simulink model "VCU_SW_2020"  (R2020b)
settings: Solver=FixedStepDiscrete  StartTime=0.0  StopTime=inf  FixedStep=1e-2  RelTol=1e-3
PreLoadFcn:
  | RTWConfigurationCB('preloadfcn', bdroot);
InitFcn:
  | loadvar_ttc500
undefined symbols (not defined in the file): BrkPedalTypes, CabMovModeTypes, cFuseTempSensAcc_X, cFuseTempSensAcc_Y, cFuseTempSensVal_X, cFuseTempSensVal_Y, cTMSTempSensVal_X, cTMSTempSensVal_Y, cTransferCaseSpeedRatio, diag_state, DoorsPositionTypes, dP_filter_Y, DriverOccClassSystemTypes, ErrorValueTypes, fatal_error_callback, IO_ADC_NO_RANGE, LadderStatusTypes, pAnalogCabRotSensAcc, pAnalogCabRotSensMaxVolt, pAnalogCabRotSensMinVolt, pAnalogCabRotSensRange, pAnalogCabRotSensZeroVolt, pBrkActivePress, pCabTiltSensAcc, pCabTiltSensMaxCur, pCabTiltSensMinCur, pDistanceCorrection, pECANManual_BPNEnable, pECANManual_BPNEnabler_Flag, pFilterSensAccRes, pHDirMaxDiffFrq, pHDirSensHighLvl, pHDirSensLowLvl, pMainGearRatio, pMaxFilterSensRes, pMaxFirstPedalSensValue, pMaxFuseTempSensRes, pMaxPressLoss, pMaxPressSensCurrent, pMaxPressValue, pMaxPressValueHydMotAndPump, pMaxPressValueParkDrain, pMaxSecondPedalSensValue, pMaxTempSensVoltage, pMaxTempValue, pMaxTMSTempSensRes, pMinFilterSensRes, pMinFirstPedalSensValue, pMinFuseTempSensRes, pMinPressLoss, pMinPressSensCurrent, pMinPressValue, pMinSecondPedalSensValue, pMinTempSensVoltage, pMinTempValue, pMinTMSTempSensRes, pMotorRingTeethNum, pPedalSensAccuracyPct, pPedalSensAccuracyVolt, pPressLossTreshhold ... (+20)
libraries: TTlibrary x270, canmsglib x127, simulink x88
(part 3 of 17)

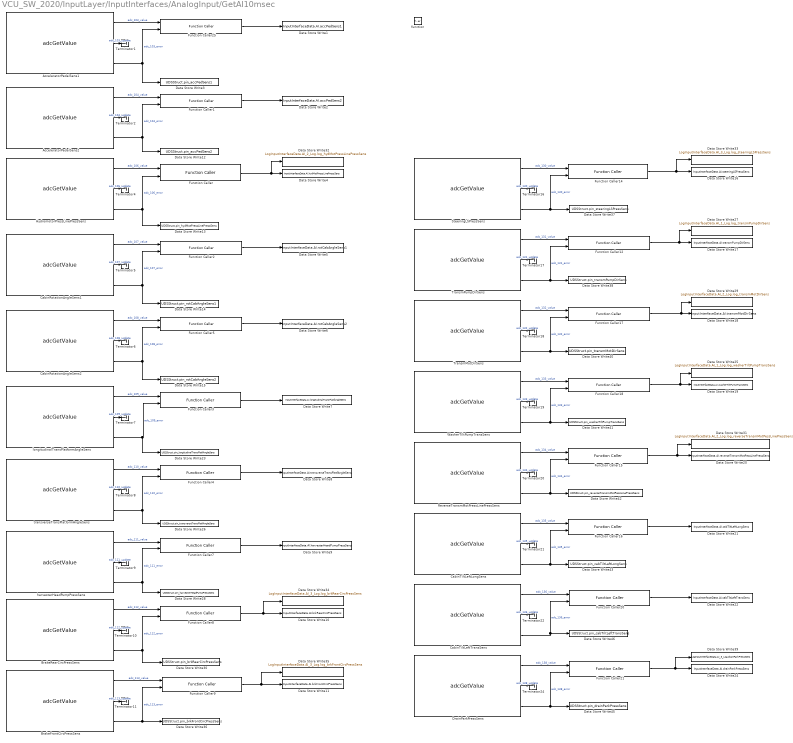
== system VCU_SW_2020/InputLayer/InputInterfaces/AnalogInput/GetAI10msec ==
  function : TriggerPort  TriggerType=function-call  VariantControl=Variant
  AcceleratorPedalSens1 : TTlibrary/ADC/adcGetValue  adc_channel=IO_ADC_00  types=IO_ADC_RATIOMETRIC  range=IO_ADC_NO_RANGE  pupd=IO_ADC_NO_PULL  sensor_supply=IO_SENSOR_SUPPLY_1  safety_conf=off  adc_val_lower=4  adc_val_upper=4  redundant_channel=IO_ADC_08  io_error=on  sample_time=-1
      settings: SourceProductName=TT control 500 series
  AcceleratorPedalSens2 : TTlibrary/ADC/adcGetValue  adc_channel=IO_ADC_02  types=IO_ADC_RATIOMETRIC  range=IO_ADC_NO_RANGE  pupd=IO_ADC_NO_PULL  sensor_supply=IO_SENSOR_SUPPLY_1  safety_conf=off  adc_val_lower=4  adc_val_upper=4  redundant_channel=IO_ADC_08  io_error=on  sample_time=-1
      settings: SourceProductName=TT control 500 series
  BrakeFrontCircPressSens : TTlibrary/ADC/adcGetValue  adc_channel=IO_ADC_20  types=IO_ADC_CURRENT  range=IO_ADC_NO_RANGE  pupd=IO_ADC_NO_PULL  sensor_supply=IO_PIN_NONE  safety_conf=off  adc_val_lower=4  adc_val_upper=4  redundant_channel=IO_ADC_08  io_error=on  sample_time=-1
      settings: SourceProductName=TT control 500 series
  BrakeRearCircPressSens : TTlibrary/ADC/adcGetValue  adc_channel=IO_ADC_18  types=IO_ADC_CURRENT  range=IO_ADC_NO_RANGE  pupd=IO_ADC_NO_PULL  sensor_supply=IO_PIN_NONE  safety_conf=off  adc_val_lower=4  adc_val_upper=4  redundant_channel=IO_ADC_08  io_error=on  sample_time=-1
      settings: SourceProductName=TT control 500 series
  CabinRotationAngleSens1 : TTlibrary/ADC/adcGetValue  adc_channel=IO_ADC_08  types=IO_ADC_RATIOMETRIC  range=IO_ADC_RANGE_5V  pupd=IO_ADC_NO_PULL  sensor_supply=IO_SENSOR_SUPPLY_2  safety_conf=off  adc_val_lower=4  adc_val_upper=4  redundant_channel=IO_ADC_08  io_error=on  sample_time=-1
      settings: SourceProductName=TT control 500 series
  CabinRotationAngleSens2 : TTlibrary/ADC/adcGetValue  adc_channel=IO_ADC_10  types=IO_ADC_RATIOMETRIC  range=IO_ADC_RANGE_5V  pupd=IO_ADC_NO_PULL  sensor_supply=IO_SENSOR_SUPPLY_2  safety_conf=off  adc_val_lower=4  adc_val_upper=4  redundant_channel=IO_ADC_08  io_error=on  sample_time=-1
      settings: SourceProductName=TT control 500 series
  CabinTiltLeftLongSens : TTlibrary/ADC/adcGetValue  adc_channel=IO_ADC_17  types=IO_ADC_CURRENT  range=IO_ADC_NO_RANGE  pupd=IO_ADC_NO_PULL  sensor_supply=IO_PIN_NONE  safety_conf=off  adc_val_lower=4  adc_val_upper=4  redundant_channel=IO_ADC_08  io_error=on  sample_time=-1
      settings: SourceProductName=TT control 500 series
  CabinTiltLeftTransSens : TTlibrary/ADC/adcGetValue  adc_channel=IO_ADC_19  types=IO_ADC_CURRENT  range=IO_ADC_NO_RANGE  pupd=IO_ADC_NO_PULL  sensor_supply=IO_PIN_NONE  safety_conf=off  adc_val_lower=4  adc_val_upper=4  redundant_channel=IO_ADC_08  io_error=on  sample_time=-1
      settings: SourceProductName=TT control 500 series
  Data Store Write1 : DataStoreWrite  DataStoreName=InputInterfaceData  DataStoreElements=InputInterfaceData.AI.accPedSens1
  Data Store Write10 : DataStoreWrite  DataStoreName=InputInterfaceData  DataStoreElements=InputInterfaceData.AI.brkRearCircPressSens
  Data Store Write11 : DataStoreWrite  DataStoreName=InputInterfaceData  DataStoreElements=InputInterfaceData.AI.brkFrontCircPressSens
  Data Store Write12 : DataStoreWrite  DataStoreName=UDSStruct  DataStoreElements=UDSStruct.pin_accPedSens2
  Data Store Write13 : DataStoreWrite  DataStoreName=UDSStruct  DataStoreElements=UDSStruct.pin_hydMotPressLinePressSens
  Data Store Write14 : DataStoreWrite  DataStoreName=UDSStruct  DataStoreElements=UDSStruct.pin_rotCabAngleSens1
  Data Store Write15 : DataStoreWrite  DataStoreName=UDSStruct  DataStoreElements=UDSStruct.pin_rotCabAngleSens2
  Data Store Write16 : DataStoreWrite  DataStoreName=InputInterfaceData  DataStoreElements=InputInterfaceData.AI.steeringLSPressSens
  Data Store Write17 : DataStoreWrite  DataStoreName=InputInterfaceData  DataStoreElements=InputInterfaceData.AI.transmPumpDirSens
  Data Store Write18 : DataStoreWrite  DataStoreName=InputInterfaceData  DataStoreElements=InputInterfaceData.AI.transmMotDirSens
  Data Store Write19 : DataStoreWrite  DataStoreName=InputInterfaceData  DataStoreElements=InputInterfaceData.AI.washerTiltPumpTransSens
  Data Store Write2 : DataStoreWrite  DataStoreName=InputInterfaceData  DataStoreElements=InputInterfaceData.AI.accPedSens2
  Data Store Write20 : DataStoreWrite  DataStoreName=InputInterfaceData  DataStoreElements=InputInterfaceData.AI.reverseTransmMotPessLinePressSens
  Data Store Write21 : DataStoreWrite  DataStoreName=InputInterfaceData  DataStoreElements=InputInterfaceData.AI.cabTiltLeftLongSens
  Data Store Write22 : DataStoreWrite  DataStoreName=InputInterfaceData  DataStoreElements=InputInterfaceData.AI.cabTiltLeftTransSens
  Data Store Write23 : DataStoreWrite  DataStoreName=UDSStruct  DataStoreElements=UDSStruct.pin_longitudinalTransPlatfAngleSens
  Data Store Write24 : DataStoreWrite  DataStoreName=InputInterfaceData  DataStoreElements=InputInterfaceData.AI.drainParkPressSens
  Data Store Write25 : DataStoreWrite  DataStoreName=LogInputInterfaceData  DataStoreElements=LogInputInterfaceData.AI_1_Log.log_washerTiltPumpTransSens
  Data Store Write26 : DataStoreWrite  DataStoreName=UDSStruct  DataStoreElements=UDSStruct.pin_transverseTransPlatfAngleSens
  Data Store Write27 : DataStoreWrite  DataStoreName=LogInputInterfaceData  DataStoreElements=LogInputInterfaceData.AI_1_Log.log_transmPumpDirSens
  Data Store Write28 : DataStoreWrite  DataStoreName=UDSStruct  DataStoreElements=UDSStruct.pin_harvesterHeadPumpPressSens
  Data Store Write29 : DataStoreWrite  DataStoreName=LogInputInterfaceData  DataStoreElements=LogInputInterfaceData.AI_2_Log.log_transmMotDirSens
  Data Store Write3 : DataStoreWrite  DataStoreName=UDSStruct  DataStoreElements=UDSStruct.pin_accPedSens1
  Data Store Write30 : DataStoreWrite  DataStoreName=UDSStruct  DataStoreElements=UDSStruct.pin_brkRearCircPressSens
  Data Store Write31 : DataStoreWrite  DataStoreName=LogInputInterfaceData  DataStoreElements=LogInputInterfaceData.AI_2_Log.log_reverseTransmMotPessLinePressSens
  Data Store Write32 : DataStoreWrite  DataStoreName=LogInputInterfaceData  DataStoreElements=LogInputInterfaceData.AI_2_Log.log_hydMotPressLinePressSens
  Data Store Write33 : DataStoreWrite  DataStoreName=LogInputInterfaceData  DataStoreElements=LogInputInterfaceData.AI_3_Log.log_steeringLSPressSens
  Data Store Write34 : DataStoreWrite  DataStoreName=LogInputInterfaceData  DataStoreElements=LogInputInterfaceData.AI_3_Log.log_brkRearCircPressSens
  Data Store Write35 : DataStoreWrite  DataStoreName=LogInputInterfaceData  DataStoreElements=LogInputInterfaceData.AI_3_Log.log_brkFrontCircPressSens
  Data Store Write36 : DataStoreWrite  DataStoreName=UDSStruct  DataStoreElements=UDSStruct.pin_brkFrontCircPressSens
  Data Store Write37 : DataStoreWrite  DataStoreName=UDSStruct  DataStoreElements=UDSStruct.pin_steeringLSPressSens
  Data Store Write38 : DataStoreWrite  DataStoreName=UDSStruct  DataStoreElements=UDSStruct.pin_transmPumpDirSens
  Data Store Write39 : DataStoreWrite  DataStoreName=LogInputInterfaceData  DataStoreElements=LogInputInterfaceData.AI_3_Log.drainParkPressSens
  Data Store Write4 : DataStoreWrite  DataStoreName=InputInterfaceData  DataStoreElements=InputInterfaceData.AI.hydMotPressLinePressSens
  Data Store Write40 : DataStoreWrite  DataStoreName=UDSStruct  DataStoreElements=UDSStruct.pin_transmMotDirSens
  Data Store Write41 : DataStoreWrite  DataStoreName=UDSStruct  DataStoreElements=UDSStruct.pin_washerTiltPumpTransSens
  Data Store Write42 : DataStoreWrite  DataStoreName=UDSStruct  DataStoreElements=UDSStruct.pin_reverseTransmMotPessLinePressSens
  Data Store Write43 : DataStoreWrite  DataStoreName=UDSStruct  DataStoreElements=UDSStruct.pin_cabTiltLeftLongSens
  Data Store Write45 : DataStoreWrite  DataStoreName=UDSStruct  DataStoreElements=UDSStruct.pin_drainParkPressSens
  Data Store Write46 : DataStoreWrite  DataStoreName=UDSStruct  DataStoreElements=UDSStruct.pin_cabTiltLeftTransSens
  Data Store Write5 : DataStoreWrite  DataStoreName=InputInterfaceData  DataStoreElements=InputInterfaceData.AI.rotCabAngleSens1
  Data Store Write6 : DataStoreWrite  DataStoreName=InputInterfaceData  DataStoreElements=InputInterfaceData.AI.rotCabAngleSens2
  Data Store Write7 : DataStoreWrite  DataStoreName=InputInterfaceData  DataStoreElements=InputInterfaceData.AI.longitudinalTransPlatfAngleSens
  Data Store Write8 : DataStoreWrite  DataStoreName=InputInterfaceData  DataStoreElements=InputInterfaceData.AI.transverseTransPlatfAngleSens
  Data Store Write9 : DataStoreWrite  DataStoreName=InputInterfaceData  DataStoreElements=InputInterfaceData.AI.harvesterHeadPumpPressSens
  DrainParkPressSens : TTlibrary/ADC/adcGetValue  adc_channel=IO_ADC_23  types=IO_ADC_CURRENT  range=IO_ADC_NO_RANGE  pupd=IO_ADC_NO_PULL  sensor_supply=IO_PIN_NONE  safety_conf=off  adc_val_lower=4  adc_val_upper=4  redundant_channel=IO_ADC_08  io_error=on  sample_time=-1
      settings: SourceProductName=TT control 500 series
  Function Caller{,3..4,7..9,14..16,20..21} (11 alike) : FunctionCaller  FunctionPrototype=finalValue = convAICurrentData(rawValue,errorSts)  InputArgumentSpecifications=<Enter example>  OutputArgumentSpecifications=<Enter example>
  Function Caller{1..2,5,12,17..18,25} (7 alike) : FunctionCaller  FunctionPrototype=finalValue = convAIVoltageData(rawValue,errorSts)  InputArgumentSpecifications=<Enter example>  OutputArgumentSpecifications=<Enter example>
  HydromotorPressLinePressSens : TTlibrary/ADC/adcGetValue  adc_channel=IO_ADC_06  types=IO_ADC_CURRENT  range=IO_ADC_NO_RANGE  pupd=IO_ADC_NO_PULL  sensor_supply=IO_PIN_NONE  safety_conf=off  adc_val_lower=4  adc_val_upper=4  redundant_channel=IO_ADC_08  io_error=on  sample_time=-1
      settings: SourceProductName=TT control 500 series
  ReverseTransmMotPressLinePressSens : TTlibrary/ADC/adcGetValue  adc_channel=IO_ADC_15  types=IO_ADC_CURRENT  range=IO_ADC_NO_RANGE  pupd=IO_ADC_NO_PULL  sensor_supply=IO_PIN_NONE  safety_conf=off  adc_val_lower=4  adc_val_upper=4  redundant_channel=IO_ADC_08  io_error=on  sample_time=-1
      settings: SourceProductName=TT control 500 series
  SteeringLSPressSens : TTlibrary/ADC/adcGetValue  adc_channel=IO_ADC_07  types=IO_ADC_CURRENT  range=IO_ADC_NO_RANGE  pupd=IO_ADC_NO_PULL  sensor_supply=IO_PIN_NONE  safety_conf=off  adc_val_lower=4  adc_val_upper=4  redundant_channel=IO_ADC_08  io_error=on  sample_time=-1
      settings: SourceProductName=TT control 500 series
  Terminator{1..2,4..11,16..22,24} (18 alike) : Terminator
  TransmMotDirSens : TTlibrary/ADC/adcGetValue  adc_channel=IO_ADC_11  types=IO_ADC_RATIOMETRIC  range=IO_ADC_RANGE_5V  pupd=IO_ADC_NO_PULL  sensor_supply=IO_PIN_NONE  safety_conf=off  adc_val_lower=4  adc_val_upper=4  redundant_channel=IO_ADC_08  io_error=on  sample_time=-1
      settings: SourceProductName=TT control 500 series
  TransmPumpDirSens : TTlibrary/ADC/adcGetValue  adc_channel=IO_ADC_09  types=IO_ADC_RATIOMETRIC  range=IO_ADC_RANGE_5V  pupd=IO_ADC_NO_PULL  sensor_supply=IO_PIN_NONE  safety_conf=off  adc_val_lower=4  adc_val_upper=4  redundant_channel=IO_ADC_08  io_error=on  sample_time=-1
      settings: SourceProductName=TT control 500 series
  WasherTiltPumpTransSens : TTlibrary/ADC/adcGetValue  adc_channel=IO_ADC_13  types=IO_ADC_RATIOMETRIC  range=IO_ADC_RANGE_5V  pupd=IO_ADC_NO_PULL  sensor_supply=IO_SENSOR_SUPPLY_0  safety_conf=off  adc_val_lower=4  adc_val_upper=4  redundant_channel=IO_ADC_08  io_error=on  sample_time=-1
      settings: SourceProductName=TT control 500 series
  harvesterHeadPumpPressSens : TTlibrary/ADC/adcGetValue  adc_channel=IO_ADC_16  types=IO_ADC_CURRENT  range=IO_ADC_NO_RANGE  pupd=IO_ADC_NO_PULL  sensor_supply=IO_PIN_NONE  safety_conf=off  adc_val_lower=4  adc_val_upper=4  redundant_channel=IO_ADC_08  io_error=on  sample_time=-1
      settings: SourceProductName=TT control 500 series
  longitudinalTransPlatformAngleSens : TTlibrary/ADC/adcGetValue  adc_channel=IO_ADC_12  types=IO_ADC_CURRENT  range=IO_ADC_NO_RANGE  pupd=IO_ADC_NO_PULL  sensor_supply=IO_PIN_NONE  safety_conf=off  adc_val_lower=4  adc_val_upper=4  redundant_channel=IO_ADC_08  io_error=on  sample_time=-1
      settings: SourceProductName=TT control 500 series
  transverseTransPlatformAngleSens : TTlibrary/ADC/adcGetValue  adc_channel=IO_ADC_14  types=IO_ADC_CURRENT  range=IO_ADC_NO_RANGE  pupd=IO_ADC_NO_PULL  sensor_supply=IO_PIN_NONE  safety_conf=off  adc_val_lower=4  adc_val_upper=4  redundant_channel=IO_ADC_08  io_error=on  sample_time=-1
      settings: SourceProductName=TT control 500 series
  wires:
  Function Caller15/1 -> Data Store Write31/1, Data Store Write20/1
  AcceleratorPedalSens1/1 -> Function Caller25/1  "adc_103_value"
  Function Caller25/1 -> Data Store Write1/1
  AcceleratorPedalSens1/3 -> Data Store Write3/1, Function Caller25/2  "adc_103_error"
  AcceleratorPedalSens1/2 -> Terminator1/1  "adc_103_update"
  AcceleratorPedalSens2/1 -> Function Caller1/1  "adc_104_value"
  Function Caller1/1 -> Data Store Write2/1
  AcceleratorPedalSens2/3 -> Function Caller1/2, Data Store Write12/1  "adc_104_error"
  AcceleratorPedalSens2/2 -> Terminator2/1  "adc_104_update"
  HydromotorPressLinePressSens/1 -> Function Caller/1  "adc_106_value"
  Function Caller/1 -> Data Store Write32/1, Data Store Write4/1
  HydromotorPressLinePressSens/3 -> Data Store Write13/1, Function Caller/2  "adc_106_error"
  HydromotorPressLinePressSens/2 -> Terminator4/1  "adc_106_update"
  CabinRotationAngleSens1/1 -> Function Caller2/1  "adc_107_value"
  Function Caller2/1 -> Data Store Write5/1
  CabinRotationAngleSens1/3 -> Data Store Write14/1, Function Caller2/2  "adc_107_error"
  CabinRotationAngleSens1/2 -> Terminator5/1  "adc_107_update"
  CabinRotationAngleSens2/1 -> Function Caller5/1  "adc_108_value"
  Function Caller5/1 -> Data Store Write6/1
  CabinRotationAngleSens2/3 -> Data Store Write15/1, Function Caller5/2  "adc_108_error"
  CabinRotationAngleSens2/2 -> Terminator6/1  "adc_108_update"
  longitudinalTransPlatformAngleSens/1 -> Function Caller3/1  "adc_109_value"
  Function Caller3/1 -> Data Store Write7/1
  longitudinalTransPlatformAngleSens/3 -> Data Store Write23/1, Function Caller3/2  "adc_109_error"
  longitudinalTransPlatformAngleSens/2 -> Terminator7/1  "adc_109_update"
  transverseTransPlatformAngleSens/1 -> Function Caller4/1  "adc_110_value"
  Function Caller4/1 -> Data Store Write8/1
  transverseTransPlatformAngleSens/3 -> Function Caller4/2, Data Store Write26/1  "adc_110_error"
  transverseTransPlatformAngleSens/2 -> Terminator8/1  "adc_110_update"
  harvesterHeadPumpPressSens/1 -> Function Caller7/1  "adc_111_value"
  Function Caller7/1 -> Data Store Write9/1
  harvesterHeadPumpPressSens/3 -> Data Store Write28/1, Function Caller7/2  "adc_111_error"
  harvesterHeadPumpPressSens/2 -> Terminator9/1  "adc_111_update"
  BrakeRearCircPressSens/1 -> Function Caller8/1  "adc_112_value"
  Function Caller8/1 -> Data Store Write34/1, Data Store Write10/1
  BrakeRearCircPressSens/3 -> Data Store Write30/1, Function Caller8/2  "adc_112_error"
  BrakeRearCircPressSens/2 -> Terminator10/1  "adc_112_update"
  BrakeFrontCircPressSens/1 -> Function Caller9/1  "adc_113_value"
  BrakeFrontCircPressSens/3 -> Data Store Write36/1, Function Caller9/2  "adc_113_error"
  BrakeFrontCircPressSens/2 -> Terminator11/1  "adc_113_update"
  SteeringLSPressSens/1 -> Function Caller14/1  "adc_130_value"
  Function Caller14/1 -> Data Store Write33/1, Data Store Write16/1
  SteeringLSPressSens/3 -> Function Caller14/2, Data Store Write37/1  "adc_130_error"
  SteeringLSPressSens/2 -> Terminator16/1  "adc_130_update"
  TransmPumpDirSens/1 -> Function Caller12/1  "adc_131_value"
  Function Caller12/1 -> Data Store Write27/1, Data Store Write17/1
  TransmPumpDirSens/3 -> Function Caller12/2, Data Store Write38/1  "adc_131_error"
  TransmPumpDirSens/2 -> Terminator17/1  "adc_131_update"
  TransmMotDirSens/1 -> Function Caller17/1  "adc_132_value"
  Function Caller17/1 -> Data Store Write29/1, Data Store Write18/1
  TransmMotDirSens/3 -> Data Store Write40/1, Function Caller17/2  "adc_132_error"
  TransmMotDirSens/2 -> Terminator18/1  "adc_132_update"
  WasherTiltPumpTransSens/1 -> Function Caller18/1  "adc_133_value"
  Function Caller18/1 -> Data Store Write25/1, Data Store Write19/1
  WasherTiltPumpTransSens/3 -> Data Store Write41/1, Function Caller18/2  "adc_133_error"
  WasherTiltPumpTransSens/2 -> Terminator19/1  "adc_133_update"
  ReverseTransmMotPressLinePressSens/1 -> Function Caller15/1  "adc_134_value"
  ReverseTransmMotPressLinePressSens/3 -> Function Caller15/2, Data Store Write42/1  "adc_134_error"
  ReverseTransmMotPressLinePressSens/2 -> Terminator20/1  "adc_134_update"
  CabinTiltLeftLongSens/1 -> Function Caller16/1  "adc_135_value"
  Function Caller16/1 -> Data Store Write21/1
  CabinTiltLeftLongSens/3 -> Data Store Write43/1, Function Caller16/2  "adc_135_error"
  CabinTiltLeftLongSens/2 -> Terminator21/1  "adc_135_update"
  CabinTiltLeftTransSens/1 -> Function Caller20/1  "adc_136_value"
  Function Caller20/1 -> Data Store Write22/1
  CabinTiltLeftTransSens/3 -> Data Store Write46/1, Function Caller20/2  "adc_136_error"
  CabinTiltLeftTransSens/2 -> Terminator22/1  "adc_136_update"
  DrainParkPressSens/1 -> Function Caller21/1  "adc_138_value"
  Function Caller21/1 -> Data Store Write39/1, Data Store Write24/1
  DrainParkPressSens/3 -> Data Store Write45/1, Function Caller21/2  "adc_138_error"
  DrainParkPressSens/2 -> Terminator24/1  "adc_138_update"
  Function Caller9/1 -> Data Store Write35/1, Data Store Write11/1

== system VCU_SW_2020/InputLayer/InputInterfaces/DigitalInput/Function-Call Subsystem ==
  function : TriggerPort  TriggerType=function-call  VariantControl=Variant
  Data Store Read1 : DataStoreRead  DataStoreName=OutputInterfaceData  DataStoreElements=OutputInterfaceData.DO.extrRightCabPosSensSupply
  Data Store Read3 : DataStoreRead  DataStoreName=OutputInterfaceData  DataStoreElements=OutputInterfaceData.DO.extrLeftCabPosSensSupply
  MATLAB Function : MATLAB Function  TreatAsAtomicUnit=on
  cabRotIndSensProc : Subsystem  TreatAsAtomicUnit=on
  wires:
  MATLAB Function/1(fcncall()) -> cabRotIndSensProc/Trigger
  Data Store Read3/1 -> MATLAB Function/1(sensSupply1)
  Data Store Read1/1 -> MATLAB Function/2(sensSupply2)

== system VCU_SW_2020/InputLayer/InputInterfaces/DigitalInput/Function-Call Subsystem1 ==
  function : TriggerPort  TriggerType=function-call  VariantControl=Variant
  Data Store Read : DataStoreRead  DataStoreName=InputInterfaceData  DataStoreElements=InputInterfaceData.DI.transCaseHighGearIsActiveSens#InputInterfaceData.DI.transCaseLowGearIsActiveSens
  Data Store Write5 : DataStoreWrite  DataStoreName=InputFunctionsData  DataStoreElements=InputFunctionsData.TransCaseGetSens
  MATLAB Function : MATLAB Function  TreatAsAtomicUnit=on
  wires:
  MATLAB Function/1(state) -> Data Store Write5/1
  Data Store Read/1 -> MATLAB Function/1(HighGear)
  Data Store Read/2 -> MATLAB Function/2(LowGear)

== system VCU_SW_2020/InputLayer/InputInterfaces/DigitalInput/Function-Call Subsystem2 ==
  function : TriggerPort  TriggerType=function-call  VariantControl=Variant
  Data Store Read1 : DataStoreRead  DataStoreName=OutputInterfaceData  DataStoreElements=OutputInterfaceData.DO.extrRightCabPosSensSupply
  Enumerated Constant : simulink/Sources/Enumerated Constant  OutDataTypeStr=Enum: StateModeTypes  Value=StateModeTypes.STT_ENABLE  SampleTime=inf
  MATLAB Function : MATLAB Function  TreatAsAtomicUnit=on
  cabRotIndSensProc : Subsystem  TreatAsAtomicUnit=on
  wires:
  Data Store Read1/1 -> MATLAB Function/2(sensSupply2)
  MATLAB Function/1(fcncall()) -> cabRotIndSensProc/Trigger
  Enumerated Constant/1 -> MATLAB Function/1(sensSupply1)

== system VCU_SW_2020/InputLayer/InputInterfaces/DigitalInput/GetDI1000msec ==
  function : TriggerPort  TriggerType=function-call  VariantControl=Variant
  Data Store Write1 : DataStoreWrite  DataStoreName=UDSStruct  DataStoreElements=UDSStruct.pin_lowCenLubrOilLvl
  Data Store Write11 : DataStoreWrite  DataStoreName=InputInterfaceData  DataStoreElements=InputInterfaceData.DI.lowCenLubrOilLvl
  Data Store Write16 : DataStoreWrite  DataStoreName=UDSStruct  DataStoreElements=UDSStruct.pin_lowBrkFluidLvlSens
  Data Store Write9 : DataStoreWrite  DataStoreName=InputInterfaceData  DataStoreElements=InputInterfaceData.DI.lowBrkFluidLvlSens
  Function Caller11 : FunctionCaller  FunctionPrototype=enumValue = convDIOSttToEnum(rawValue,errorSts)  InputArgumentSpecifications=<Enter example>  OutputArgumentSpecifications=<Enter example>
  Function Caller9 : FunctionCaller  FunctionPrototype=enumValue = convDIOSttToEnum(rawValue,errorSts)  InputArgumentSpecifications=<Enter example>  OutputArgumentSpecifications=<Enter example>
  LowBrakeFluidLevelSens : TTlibrary/DIO/getDigitalInputValue  di_channel=IO_DI_41  pupd=IO_DI_PD_10K  limits=off  low_thresh1=0  low_thresh2=2500  high_thresh1=2500  high_thresh2=32000  io_error=on  sample_time=-1
      settings: SourceProductName=TT control 500 series
  LowCenLubrOilLevel : TTlibrary/DIO/getDigitalInputValue  di_channel=IO_DI_45  pupd=IO_DI_PD_10K  limits=off  low_thresh1=0  low_thresh2=2500  high_thresh1=2500  high_thresh2=32000  io_error=on  sample_time=-1
      settings: SourceProductName=TT control 500 series
  wires:
  Function Caller11/1 -> Data Store Write11/1
  LowCenLubrOilLevel/1 -> Function Caller11/1  "di_147_value"
  LowCenLubrOilLevel/2 -> Data Store Write1/1, Function Caller11/2  "di_147_error"
  LowBrakeFluidLevelSens/2 -> Data Store Write16/1, Function Caller9/2  "di_141_error"
  Function Caller9/1 -> Data Store Write9/1
  LowBrakeFluidLevelSens/1 -> Function Caller9/1  "di_141_value"

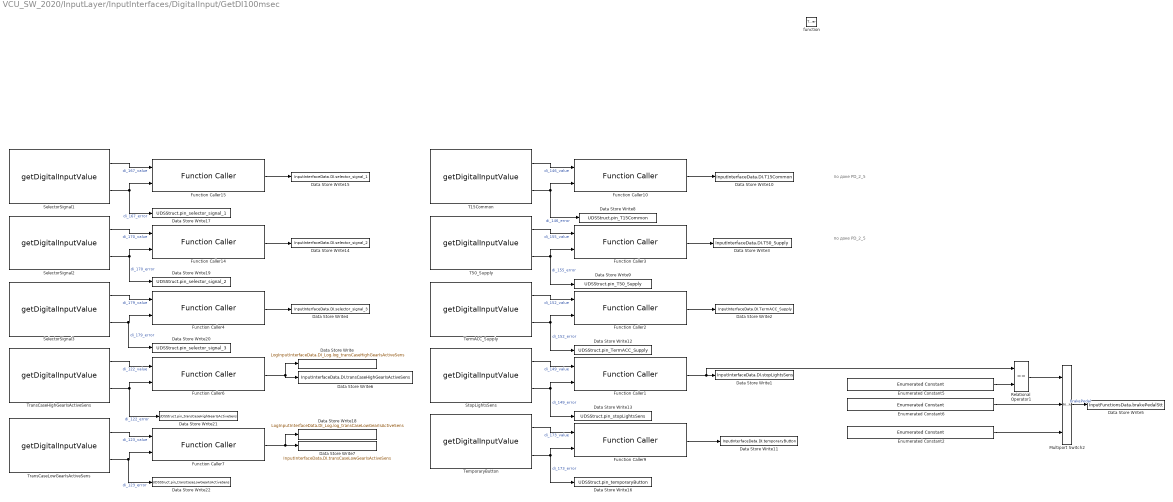
== system VCU_SW_2020/InputLayer/InputInterfaces/DigitalInput/GetDI100msec ==
  note: по доке PD_2_5
  note: по доке PD_2_5
  function : TriggerPort  TriggerType=function-call  VariantControl=Variant
  Data Store Write : DataStoreWrite  DataStoreName=LogInputInterfaceData  DataStoreElements=LogInputInterfaceData.DI_Log.log_transCaseHighGearIsActiveSens
  Data Store Write1 : DataStoreWrite  DataStoreName=InputInterfaceData  DataStoreElements=InputInterfaceData.DI.stopLightsSens
  Data Store Write10 : DataStoreWrite  DataStoreName=InputInterfaceData  DataStoreElements=InputInterfaceData.DI.T15Common
  Data Store Write11 : DataStoreWrite  DataStoreName=InputInterfaceData  DataStoreElements=InputInterfaceData.DI.temporaryButton
  Data Store Write12 : DataStoreWrite  DataStoreName=UDSStruct  DataStoreElements=UDSStruct.pin_TermACC_Supply
  Data Store Write13 : DataStoreWrite  DataStoreName=UDSStruct  DataStoreElements=UDSStruct.pin_stopLightsSens
  Data Store Write14 : DataStoreWrite  DataStoreName=InputInterfaceData  DataStoreElements=InputInterfaceData.DI.selector_signal_2
  Data Store Write15 : DataStoreWrite  DataStoreName=InputInterfaceData  DataStoreElements=InputInterfaceData.DI.selector_signal_1
  Data Store Write16 : DataStoreWrite  DataStoreName=UDSStruct  DataStoreElements=UDSStruct.pin_temporaryButton
  Data Store Write17 : DataStoreWrite  DataStoreName=UDSStruct  DataStoreElements=UDSStruct.pin_selector_signal_1
  Data Store Write18 : DataStoreWrite  DataStoreName=LogInputInterfaceData  DataStoreElements=LogInputInterfaceData.DI_Log.log_transCaseLowGearIsActiveSens
  Data Store Write19 : DataStoreWrite  DataStoreName=UDSStruct  DataStoreElements=UDSStruct.pin_selector_signal_2
  Data Store Write2 : DataStoreWrite  DataStoreName=InputInterfaceData  DataStoreElements=InputInterfaceData.DI.TermACC_Supply
  Data Store Write20 : DataStoreWrite  DataStoreName=UDSStruct  DataStoreElements=UDSStruct.pin_selector_signal_3
  Data Store Write21 : DataStoreWrite  DataStoreName=UDSStruct  DataStoreElements=UDSStruct.pin_transCaseHighGearIsActiveSens
  Data Store Write22 : DataStoreWrite  DataStoreName=UDSStruct  DataStoreElements=UDSStruct.pin_transCaseLowGearIsActiveSens
  Data Store Write3 : DataStoreWrite  DataStoreName=InputInterfaceData  DataStoreElements=InputInterfaceData.DI.T50_Supply
  Data Store Write4 : DataStoreWrite  DataStoreName=InputInterfaceData  DataStoreElements=InputInterfaceData.DI.selector_signal_3
  Data Store Write5 : DataStoreWrite  DataStoreName=InputFunctionsData  DataStoreElements=InputFunctionsData.brakePedalStt
  Data Store Write6 : DataStoreWrite  DataStoreName=InputInterfaceData  DataStoreElements=InputInterfaceData.DI.transCaseHighGearIsActiveSens
  Data Store Write7 : DataStoreWrite  DataStoreName=InputInterfaceData  DataStoreElements=InputInterfaceData.DI.transCaseLowGearIsActiveSens
  Data Store Write8 : DataStoreWrite  DataStoreName=UDSStruct  DataStoreElements=UDSStruct.pin_T15Common
  Data Store Write9 : DataStoreWrite  DataStoreName=UDSStruct  DataStoreElements=UDSStruct.pin_T50_Supply
  Enumerated Constant2 : simulink/Sources/Enumerated Constant  OutDataTypeStr=Enum: BrkPedalTypes  Value=BrkPedalTypes.BRK_PED_PRESSED  SampleTime=inf
  Enumerated Constant5 : simulink/Sources/Enumerated Constant  OutDataTypeStr=Enum: StateModeTypes  Value=StateModeTypes.STT_ENABLE  SampleTime=inf
  Enumerated Constant6 : simulink/Sources/Enumerated Constant  OutDataTypeStr=Enum: BrkPedalTypes  Value=BrkPedalTypes.BRK_PED_RELEASED  SampleTime=inf
  Function Caller{1..4,6..7,9..10,14..15} (10 alike) : FunctionCaller  FunctionPrototype=enumValue = convDIOSttToEnum(rawValue,errorSts)  InputArgumentSpecifications=<Enter example>  OutputArgumentSpecifications=<Enter example>
  Multiport Switch2 : MultiPortSwitch  DataPortOrder=Zero-based contiguous  Inputs=2  zeroidx=on
  Relational Operator1 : RelationalOperator  Operator===  OutDataTypeStr=boolean  RndMeth=Simplest
  SelectorSignal1 : TTlibrary/DIO/getDigitalInputValue  di_channel=IO_DI_93  pupd=IO_DI_PD_10K  limits=off  low_thresh1=0  low_thresh2=2500  high_thresh1=2500  high_thresh2=32000  io_error=on  sample_time=-1
      settings: SourceProductName=TT control 500 series
  SelectorSignal2 : TTlibrary/DIO/getDigitalInputValue  di_channel=IO_DI_95  pupd=IO_DI_PD_10K  limits=off  low_thresh1=0  low_thresh2=2500  high_thresh1=2500  high_thresh2=32000  io_error=on  sample_time=-1
      settings: SourceProductName=TT control 500 series
  SelectorSignal3 : TTlibrary/DIO/getDigitalInputValue  di_channel=IO_DI_77  pupd=IO_DI_PD_10K  limits=off  low_thresh1=0  low_thresh2=2500  high_thresh1=2500  high_thresh2=32000  io_error=on  sample_time=-1
      settings: SourceProductName=TT control 500 series
  StopLightsSens : TTlibrary/DIO/getDigitalInputValue  di_channel=IO_DI_72  pupd=IO_DI_PD_10K  limits=off  low_thresh1=0  low_thresh2=2500  high_thresh1=2500  high_thresh2=32000  io_error=on  sample_time=-1
      settings: SourceProductName=TT control 500 series
  T15Common : TTlibrary/DIO/getDigitalInputValue  di_channel=IO_DI_43  pupd=IO_DI_PD_10K  limits=off  low_thresh1=0  low_thresh2=2500  high_thresh1=2500  high_thresh2=32000  io_error=on  sample_time=-1
      settings: SourceProductName=TT control 500 series
  T50_Supply : TTlibrary/DIO/getDigitalInputValue  di_channel=IO_DI_76  pupd=IO_DI_PD_10K  limits=off  low_thresh1=0  low_thresh2=2500  high_thresh1=2500  high_thresh2=32000  io_error=on  sample_time=-1
      settings: SourceProductName=TT control 500 series
  TemporaryButton : TTlibrary/DIO/getDigitalInputValue  di_channel=IO_DI_73  pupd=IO_DI_PD_10K  limits=off  low_thresh1=0  low_thresh2=2500  high_thresh1=2500  high_thresh2=32000  io_error=on  sample_time=-1
      settings: SourceProductName=TT control 500 series
  TermACC_Supply : TTlibrary/DIO/getDigitalInputValue  di_channel=IO_DI_74  pupd=IO_DI_PD_10K  limits=off  low_thresh1=0  low_thresh2=2500  high_thresh1=2500  high_thresh2=32000  io_error=on  sample_time=-1
      settings: SourceProductName=TT control 500 series
  TransCaseHighGearIsActiveSens : TTlibrary/DIO/getDigitalInputValue  di_channel=IO_DI_42  pupd=IO_DI_PD_10K  limits=off  low_thresh1=0  low_thresh2=2500  high_thresh1=2500  high_thresh2=32000  io_error=on  sample_time=-1
      settings: SourceProductName=TT control 500 series
  TransCaseLowGearIsActiveSens : TTlibrary/DIO/getDigitalInputValue  di_channel=IO_DI_44  pupd=IO_DI_PD_10K  limits=off  low_thresh1=0  low_thresh2=2500  high_thresh1=2500  high_thresh2=32000  io_error=on  sample_time=-1
      settings: SourceProductName=TT control 500 series
  wires:
  TemporaryButton/1 -> Function Caller9/1  "di_173_value"
  TemporaryButton/2 -> Data Store Write16/1, Function Caller9/2  "di_173_error"
  Function Caller9/1 -> Data Store Write11/1
  StopLightsSens/2 -> Data Store Write13/1, Function Caller1/2  "di_149_error"
  StopLightsSens/1 -> Function Caller1/1  "di_149_value"
  TransCaseLowGearIsActiveSens/2 -> Data Store Write22/1, Function Caller7/2  "di_123_error"
  Function Caller7/1 -> Data Store Write7/1, Data Store Write18/1
  TransCaseLowGearIsActiveSens/1 -> Function Caller7/1  "di_123_value"
  TransCaseHighGearIsActiveSens/2 -> Data Store Write21/1, Function Caller6/2  "di_122_error"
  TransCaseHighGearIsActiveSens/1 -> Function Caller6/1  "di_122_value"
  Function Caller6/1 -> Data Store Write6/1, Data Store Write/1
  SelectorSignal3/1 -> Function Caller4/1  "di_179_value"
  Function Caller14/1 -> Data Store Write14/1
  SelectorSignal3/2 -> Data Store Write20/1, Function Caller4/2  "di_179_error"
  Function Caller4/1 -> Data Store Write4/1
  Function Caller15/1 -> Data Store Write15/1
  SelectorSignal2/1 -> Function Caller14/1  "di_170_value"
  SelectorSignal1/2 -> Data Store Write17/1, Function Caller15/2  "di_167_error"
  SelectorSignal2/2 -> Function Caller14/2, Data Store Write19/1  "di_170_error"
  SelectorSignal1/1 -> Function Caller15/1  "di_167_value"
  Function Caller2/1 -> Data Store Write2/1
  TermACC_Supply/1 -> Function Caller2/1  "di_152_value"
  TermACC_Supply/2 -> Function Caller2/2, Data Store Write12/1  "di_152_error"
  T50_Supply/1 -> Function Caller3/1  "di_155_value"
  T50_Supply/2 -> Data Store Write9/1, Function Caller3/2  "di_155_error"
  Function Caller3/1 -> Data Store Write3/1
  T15Common/2 -> Data Store Write8/1, Function Caller10/2  "di_146_error"
  Function Caller10/1 -> Data Store Write10/1
  T15Common/1 -> Function Caller10/1  "di_146_value"
  Enumerated Constant6/1 -> Multiport Switch2/2
  Enumerated Constant2/1 -> Multiport Switch2/3
  Enumerated Constant5/1 -> Relational Operator1/2
  Function Caller1/1 -> Relational Operator1/1, Data Store Write1/1
  Relational Operator1/1 -> Multiport Switch2/1
  Multiport Switch2/1 -> Data Store Write5/1  "brakePedal"

== system VCU_SW_2020/InputLayer/InputInterfaces/DigitalInput/GetDI10msec ==
  note: по доке PD_2_5
  note: по доке PD_2_5
  function : TriggerPort  TriggerType=function-call  VariantControl=Variant
  Data Store Write : DataStoreWrite  DataStoreName=UDSStruct  DataStoreElements=UDSStruct.pin_engAirFilterClogSens
  Data Store Write1 : DataStoreWrite  DataStoreName=UDSStruct  DataStoreElements=UDSStruct.pin_extrLeftCabPosSens
  Data Store Write12 : DataStoreWrite  DataStoreName=InputInterfaceData  DataStoreElements=InputInterfaceData.DI.shutdownButtonSig
  Data Store Write16 : DataStoreWrite  DataStoreName=InputInterfaceData  DataStoreElements=InputInterfaceData.DI.extrLeftCabPosSens
  Data Store Write17 : DataStoreWrite  DataStoreName=InputInterfaceData  DataStoreElements=InputInterfaceData.DI.extrRightCabPosSens
  Data Store Write19 : DataStoreWrite  DataStoreName=LogInputInterfaceData  DataStoreElements=LogInputInterfaceData.DI_Log.log_shutdownButtonSig
  Data Store Write2 : DataStoreWrite  DataStoreName=UDSStruct  DataStoreElements=UDSStruct.pin_extrRightCabPosSens
  Data Store Write3 : DataStoreWrite  DataStoreName=UDSStruct  DataStoreElements=UDSStruct.pin_shutdownButtonSig
  ExtrLeftCabPosSens : TTlibrary/DIO/getDigitalInputValue  di_channel=IO_DI_90  pupd=IO_DI_PD_10K  limits=off  low_thresh1=0  low_thresh2=2500  high_thresh1=2500  high_thresh2=32000  io_error=on  sample_time=-1
      settings: SourceProductName=TT control 500 series
  ExtrRightCabinePosSens : TTlibrary/DIO/getDigitalInputValue  di_channel=IO_DI_94  pupd=IO_DI_PD_10K  limits=off  low_thresh1=0  low_thresh2=2500  high_thresh1=2500  high_thresh2=32000  io_error=on  sample_time=-1
      settings: SourceProductName=TT control 500 series
  Function Caller12 : FunctionCaller  FunctionPrototype=enumValue = convDIOSttToEnum(rawValue,errorSts)  InputArgumentSpecifications=<Enter example>  OutputArgumentSpecifications=<Enter example>
  Function Caller16 : FunctionCaller  FunctionPrototype=enumValue = convDIOSttToEnum(rawValue,errorSts)  InputArgumentSpecifications=<Enter example>  OutputArgumentSpecifications=<Enter example>
  Function Caller17 : FunctionCaller  FunctionPrototype=enumValue = convDIOSttToEnum(rawValue,errorSts)  InputArgumentSpecifications=<Enter example>  OutputArgumentSpecifications=<Enter example>
  ShutdownButtonSig : TTlibrary/DIO/getDigitalInputValue  di_channel=IO_DI_47  pupd=IO_DI_PD_10K  limits=off  low_thresh1=0  low_thresh2=2500  high_thresh1=2500  high_thresh2=32000  io_error=on  sample_time=-1
      settings: SourceProductName=TT control 500 series
  wires:
  ExtrRightCabinePosSens/1 -> Function Caller17/1  "di_194_value"
  ExtrRightCabinePosSens/2 -> Data Store Write2/1, Function Caller17/2  "di_194_error"
  ExtrLeftCabPosSens/1 -> Function Caller16/1  "di_188_value"
  ExtrLeftCabPosSens/2 -> Data Store Write1/1, Function Caller16/2  "di_188_error"
  ShutdownButtonSig/1 -> Function Caller12/1  "di_148_value"
  Function Caller12/1 -> Data Store Write12/1, Data Store Write19/1
  ShutdownButtonSig/2 -> Data Store Write3/1, Function Caller12/2  "di_148_error"
  Function Caller16/1 -> Data Store Write16/1
  Function Caller17/1 -> Data Store Write17/1

== system VCU_SW_2020/InputLayer/InputInterfaces/PWDInput/GetPWD1000msec ==
  function : TriggerPort  TriggerType=function-call  VariantControl=Variant

== system VCU_SW_2020/InputLayer/InputInterfaces/PWDInput/GetPWD100msec ==
  function : TriggerPort  TriggerType=function-call  VariantControl=Variant
  Bus Selector : BusSelector  OutputSignals=pulse_samples_count
  Bus Selector1 : BusSelector  OutputSignals=pulse_samples_count
  Data Store Write : DataStoreWrite  DataStoreName=LogInputInterfaceData  DataStoreElements=LogInputInterfaceData.AI_1_Log.log_transPumpSpdSensSig2
  Data Store Write1 : DataStoreWrite  DataStoreName=InputInterfaceData  DataStoreElements=InputInterfaceData.PWD.transmHydMotSpdSensSig1
  Data Store Write10 : DataStoreWrite  DataStoreName=UDSStruct  DataStoreElements=UDSStruct.pin_transmHydMotSpdSensSig1
  Data Store Write11 : DataStoreWrite  DataStoreName=UDSStruct  DataStoreElements=UDSStruct.pin_transmHydMotSpdSensSig2
  Data Store Write12 : DataStoreWrite  DataStoreName=UDSStruct  DataStoreElements=UDSStruct.pin_transPumpSpdSensSig2
  Data Store Write13 : DataStoreWrite  DataStoreName=UDSStruct  DataStoreElements=UDSStruct.pin_transPumpSpdSensSig1
  Data Store Write2 : DataStoreWrite  DataStoreName=InputInterfaceData  DataStoreElements=InputInterfaceData.PWD.transmHydMotSpdSensSig2
  Data Store Write3 : DataStoreWrite  DataStoreName=InputInterfaceData  DataStoreElements=InputInterfaceData.PWD.transPumpSpdSensSig2
  Data Store Write4 : DataStoreWrite  DataStoreName=InputInterfaceData  DataStoreElements=InputInterfaceData.PWD.transPumpSpdSensSig1
  Data Store Write5 : DataStoreWrite  DataStoreName=LogInputInterfaceData  DataStoreElements=LogInputInterfaceData.AI_1_Log.log_transPumpSpdSensSig1
  Data Store Write6 : DataStoreWrite  DataStoreName=LogInputInterfaceData  DataStoreElements=LogInputInterfaceData.AI_2_Log.log_transmHydMotSpdSensSig1
  Data Store Write7 : DataStoreWrite  DataStoreName=LogInputInterfaceData  DataStoreElements=LogInputInterfaceData.AI_2_Log.log_transmHydMotSpdSensSig2
  Data Store Write8 : DataStoreWrite  DataStoreName=InputInterfaceData  DataStoreElements=InputInterfaceData.PWD.transmHydMotPulseSamples1
  Data Store Write9 : DataStoreWrite  DataStoreName=InputInterfaceData  DataStoreElements=InputInterfaceData.PWD.transmHydMotPulseSamples2
  Data Type Conversion : DataTypeConversion  OutDataTypeStr=uint16
  Data Type Conversion1 : DataTypeConversion  OutDataTypeStr=uint16
  Function Caller{,1..3} (4 alike) : FunctionCaller  FunctionPrototype=finalValue = convPWDData(rawValue,errorSts)  InputArgumentSpecifications=<Enter example>  OutputArgumentSpecifications=<Enter example>
  MATLAB Function8 : MATLAB Function  Commented=on  TreatAsAtomicUnit=on
  Terminator{,1..4,6,8..10,12} (10 alike) : Terminator
  TransPumpSpeedSensSig1 : TTlibrary/PWD/pwdComplexGet  timer_channel=IO_PWD_01  pulse_mode=IO_PWD_HIGH_TIME  freq_mode=IO_PWD_RISING_VAR  capture_count=4  pupd=IO_PWD_PD_10K  safety_conf=off  pwd_freq_val_lower=0  pwd_freq_val_upper=0  pwd_pulse_val_lower=0  pwd_pulse_val_upper=0  io_error=on  sample_time=-1
      settings: SourceProductName=TT control 500 series
  TransPumpSpeedSensSig2 : TTlibrary/PWD/pwdComplexGet  timer_channel=IO_PWD_03  pulse_mode=IO_PWD_HIGH_TIME  freq_mode=IO_PWD_RISING_VAR  capture_count=4  pupd=IO_PWD_PD_10K  safety_conf=off  pwd_freq_val_lower=0  pwd_freq_val_upper=0  pwd_pulse_val_lower=0  pwd_pulse_val_upper=0  io_error=on  sample_time=-1
      settings: SourceProductName=TT control 500 series
  TransmHydromotorSpeedAndPulseSig1 : TTlibrary/PWD/pwdComplexGet  timer_channel=IO_PWD_02  pulse_mode=IO_PWD_HIGH_TIME  freq_mode=IO_PWD_RISING_VAR  capture_count=4  pupd=IO_PWD_PD_10K  safety_conf=off  pwd_freq_val_lower=0  pwd_freq_val_upper=0  pwd_pulse_val_lower=0  pwd_pulse_val_upper=0  io_error=on  sample_time=-1
      settings: SourceProductName=TT control 500 series
  TransmHydromotorSpeedAndPulseSig2 : TTlibrary/PWD/pwdComplexGet  timer_channel=IO_PWD_04  pulse_mode=IO_PWD_HIGH_TIME  freq_mode=IO_PWD_RISING_VAR  capture_count=4  pupd=IO_PWD_PD_10K  safety_conf=off  pwd_freq_val_lower=0  pwd_freq_val_upper=0  pwd_pulse_val_lower=0  pwd_pulse_val_upper=0  io_error=on  sample_time=-1
      settings: SourceProductName=TT control 500 series
  wires:
  Data Type Conversion1/1 -> Data Store Write9/1
  TransmHydromotorSpeedAndPulseSig2/4 -> Bus Selector1/1  "io_pwd_04_samples"
  Bus Selector1/1 -> Data Type Conversion1/1  "<pulse_samples_count>"
  Data Type Conversion/1 -> Data Store Write8/1
  Bus Selector/1 -> Data Type Conversion/1  "<pulse_samples_count>"
  TransmHydromotorSpeedAndPulseSig1/4 -> Bus Selector/1  "io_pwd_02_samples"
  TransmHydromotorSpeedAndPulseSig2/1 -> Function Caller1/1  "io_pwd_04_freq_value"
  TransPumpSpeedSensSig2/1 -> Function Caller3/1  "io_pwd_03_freq_value"
  TransPumpSpeedSensSig1/1 -> Function Caller2/1  "io_pwd_01_freq_value"
  TransPumpSpeedSensSig2/4 -> Terminator10/1  "io_pwd_03_samples"
  TransPumpSpeedSensSig2/3 -> Terminator4/1  "io_pwd_03_pin_value"
  Function Caller/1 -> Data Store Write6/1, Data Store Write1/1
  TransPumpSpeedSensSig1/4 -> Terminator8/1  "io_pwd_01_samples"
  TransPumpSpeedSensSig2/2 -> Terminator9/1  "io_pwd_03_pw_value"
  TransmHydromotorSpeedAndPulseSig2/2 -> Terminator6/1  "io_pwd_04_pw_value"
  TransPumpSpeedSensSig2/5 -> Data Store Write13/1, Function Caller3/2  "io_pwd_03_error"
  Function Caller2/1 -> Data Store Write3/1, Data Store Write/1
  TransmHydromotorSpeedAndPulseSig1/5 -> Data Store Write10/1, Function Caller/2  "io_pwd_02_error"
  TransmHydromotorSpeedAndPulseSig1/1 -> Function Caller/1  "io_pwd_02_freq_value"
  TransmHydromotorSpeedAndPulseSig2/3 -> Terminator1/1  "io_pwd_04_pin_value"
  TransPumpSpeedSensSig1/2 -> Terminator3/1  "io_pwd_01_pw_value"
  TransPumpSpeedSensSig1/3 -> Terminator2/1  "io_pwd_01_pin_value"
  TransPumpSpeedSensSig1/5 -> Function Caller2/2, Data Store Write12/1  "io_pwd_01_error"
  Function Caller3/1 -> Data Store Write4/1, Data Store Write5/1
  Function Caller1/1 -> Data Store Write7/1, Data Store Write2/1
  TransmHydromotorSpeedAndPulseSig1/3 -> Terminator/1  "io_pwd_02_pin_value"
  TransmHydromotorSpeedAndPulseSig1/2 -> Terminator12/1  "io_pwd_02_pw_value"
  TransmHydromotorSpeedAndPulseSig2/5 -> Data Store Write11/1, Function Caller1/2  "io_pwd_04_error"

== system VCU_SW_2020/InputLayer/InputInterfaces/PWDInput/GetPWD10msec ==
  function : TriggerPort  TriggerType=function-call  VariantControl=Variant

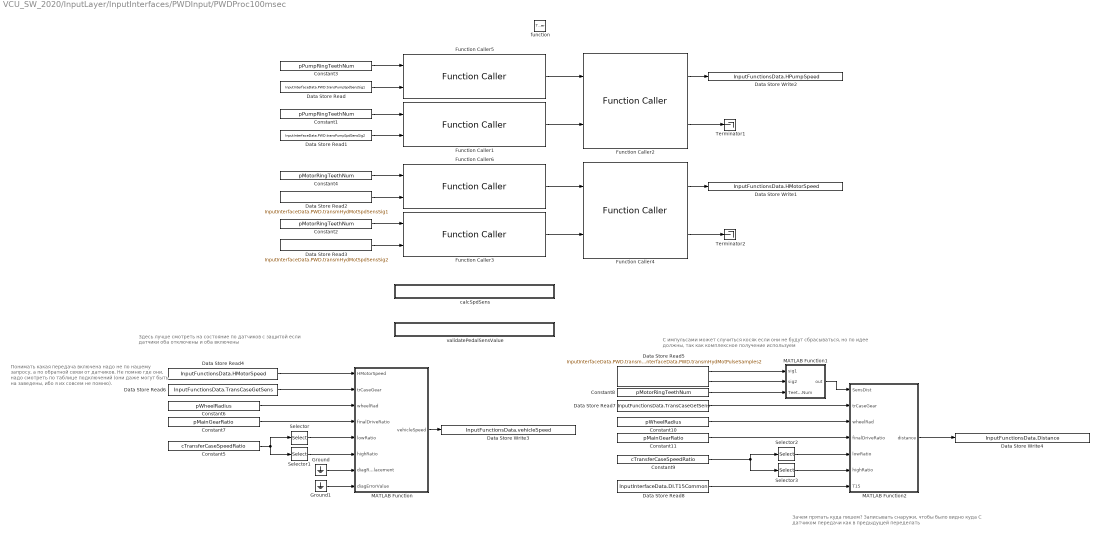
== system VCU_SW_2020/InputLayer/InputInterfaces/PWDInput/PWDProc100msec ==
  note: Понимать какая передача включена надо не по нашему запросу, а по обратной связи от датчиков.
      | Не помню где они, надо смотреть по таблице подключений (они даже могут быть на заведены, ибо я их совсем не помню).
  note: С импульсами может случиться косяк если они не будут сбрасываться, но по идее должны, так как комплексное получение используем
  note: Зачем прятать куда пишем? Записывать снаружи, чтобы было видно куда
      | С датчиком передачи как в предыдущей переделать
  note: Здесь лучше смотреть на состояние по датчиков
      | с защитой если датчики оба отключены и оба включены
  function : TriggerPort  TriggerType=function-call  VariantControl=Variant
  Constant1 : Constant  Value=pPumpRingTeethNum
  Constant10 : Constant  Value=pWheelRadius
  Constant11 : Constant  Value=pMainGearRatio
  Constant2 : Constant  Value=pMotorRingTeethNum
  Constant3 : Constant  Value=pPumpRingTeethNum
  Constant4 : Constant  Value=pMotorRingTeethNum
  Constant5 : Constant  Value=cTransferCaseSpeedRatio
  Constant6 : Constant  Value=pWheelRadius
  Constant7 : Constant  Value=pMainGearRatio
  Constant8 : Constant  Value=pMotorRingTeethNum
  Constant9 : Constant  Value=cTransferCaseSpeedRatio
  Data Store Read : DataStoreRead  DataStoreName=InputInterfaceData  DataStoreElements=InputInterfaceData.PWD.transPumpSpdSensSig1
  Data Store Read1 : DataStoreRead  DataStoreName=InputInterfaceData  DataStoreElements=InputInterfaceData.PWD.transPumpSpdSensSig2
  Data Store Read2 : DataStoreRead  DataStoreName=InputInterfaceData  DataStoreElements=InputInterfaceData.PWD.transmHydMotSpdSensSig1
  Data Store Read3 : DataStoreRead  DataStoreName=InputInterfaceData  DataStoreElements=InputInterfaceData.PWD.transmHydMotSpdSensSig2
  Data Store Read4 : DataStoreRead  DataStoreName=InputFunctionsData  DataStoreElements=InputFunctionsData.HMotorSpeed
  Data Store Read5 : DataStoreRead  DataStoreName=InputInterfaceData  DataStoreElements=InputInterfaceData.PWD.transmHydMotPulseSamples1#InputInterfaceData.PWD.transmHydMotPulseSamples2
  Data Store Read6 : DataStoreRead  DataStoreName=InputFunctionsData  DataStoreElements=InputFunctionsData.TransCaseGetSens
  Data Store Read7 : DataStoreRead  DataStoreName=InputFunctionsData  DataStoreElements=InputFunctionsData.TransCaseGetSens
  Data Store Read8 : DataStoreRead  DataStoreName=InputInterfaceData  DataStoreElements=InputInterfaceData.DI.T15Common
  Data Store Write1 : DataStoreWrite  DataStoreName=InputFunctionsData  DataStoreElements=InputFunctionsData.HMotorSpeed
  Data Store Write2 : DataStoreWrite  DataStoreName=InputFunctionsData  DataStoreElements=InputFunctionsData.HPumpSpeed
  Data Store Write3 : DataStoreWrite  DataStoreName=InputFunctionsData  DataStoreElements=InputFunctionsData.vehicleSpeed
  Data Store Write4 : DataStoreWrite  DataStoreName=InputFunctionsData  DataStoreElements=InputFunctionsData.Distance
  Function Caller{1,3,5..6} (4 alike) : FunctionCaller  FunctionPrototype=SpdValue = calcSpdSensValue(teethNum,sensFreq)  InputArgumentSpecifications=<Enter example>  OutputArgumentSpecifications=<Enter example>
  Function Caller2 : FunctionCaller  FunctionPrototype=[SpdVal,errorSts] = validateSpdSensValue(fstValue,secValue)  InputArgumentSpecifications=<Enter example>  OutputArgumentSpecifications=<Enter example>
  Function Caller4 : FunctionCaller  FunctionPrototype=[SpdVal,errorSts] = validateSpdSensValue(fstValue,secValue)  InputArgumentSpecifications=<Enter example>  OutputArgumentSpecifications=<Enter example>
  Ground : Ground
  Ground1 : Ground
  MATLAB Function : MATLAB Function  TreatAsAtomicUnit=on
  MATLAB Function1 : MATLAB Function  TreatAsAtomicUnit=on
  MATLAB Function2 : MATLAB Function  TreatAsAtomicUnit=on
  Selector : Selector  InputPortWidth=2  IndexOptions=Index vector (dialog)  Indices=2  OutputSizes=1
  Selector1 : Selector  InputPortWidth=2  IndexOptions=Index vector (dialog)  Indices=1  OutputSizes=1
  Selector2 : Selector  InputPortWidth=2  IndexOptions=Index vector (dialog)  Indices=2  OutputSizes=1
  Selector3 : Selector  InputPortWidth=2  IndexOptions=Index vector (dialog)  Indices=1  OutputSizes=1
  Terminator1 : Terminator
  Terminator2 : Terminator
  calcSpdSens : Subsystem  TreatAsAtomicUnit=on
  validatePedalSensValue : Subsystem  TreatAsAtomicUnit=on
  wires:
  Data Store Read8/1 -> MATLAB Function2/7(T15)
  Data Store Read7/1 -> MATLAB Function2/2(trCaseGear)
  MATLAB Function1/1(out) -> MATLAB Function2/1(SensDist)
  Constant10/1 -> MATLAB Function2/3(wheelRad)
  Constant11/1 -> MATLAB Function2/4(finalDriveRatio)
  Selector3/1 -> MATLAB Function2/6(highRatio)
  Selector2/1 -> MATLAB Function2/5(lowRatio)
  Constant9/1 -> Selector2/1, Selector3/1
  Constant8/1 -> MATLAB Function1/3(TeethNum)
  Data Store Read5/2 -> MATLAB Function1/2(sig2)
  Data Store Read5/1 -> MATLAB Function1/1(sig1)
  Data Store Read1/1 -> Function Caller1/2
  Data Store Read/1 -> Function Caller5/2
  Function Caller3/1 -> Function Caller4/2
  Function Caller1/1 -> Function Caller2/2
  Function Caller4/1 -> Data Store Write1/1
  Constant1/1 -> Function Caller1/1
  Constant2/1 -> Function Caller3/1
  Constant4/1 -> Function Caller6/1
  Data Store Read2/1 -> Function Caller6/2
  Data Store Read3/1 -> Function Caller3/2
  Constant3/1 -> Function Caller5/1
  Function Caller2/1 -> Data Store Write2/1
  Function Caller4/2 -> Terminator2/1
  Function Caller6/1 -> Function Caller4/1
  Function Caller5/1 -> Function Caller2/1
  Function Caller2/2 -> Terminator1/1
  MATLAB Function2/1(distance) -> Data Store Write4/1
  Constant5/1 -> Selector/1, Selector1/1
  Constant7/1 -> MATLAB Function/4(finalDriveRatio)
  Data Store Read6/1 -> MATLAB Function/2(trCaseGear)
  Selector1/1 -> MATLAB Function/6(highRatio)
  Selector/1 -> MATLAB Function/5(lowRatio)
  Data Store Read4/1 -> MATLAB Function/1(HMotorSpeed)
  Ground1/1 -> MATLAB Function/8(diagErrorValue)
  Constant6/1 -> MATLAB Function/3(wheelRad)
  Ground/1 -> MATLAB Function/7(diagReplacement)
  MATLAB Function/1(vehicleSpeed) -> Data Store Write3/1

== system VCU_SW_2020/InputLayer/InputInterfaces/PWMCurrentInput/GetPWMCur1000msec ==
  function : TriggerPort  TriggerType=function-call  VariantControl=Variant

== system VCU_SW_2020/InputLayer/InputInterfaces/PWMCurrentInput/GetPWMCur100msec ==
  function : TriggerPort  TriggerType=function-call  VariantControl=Variant
